simulink model "pend_slidingmode"  (Simulink 9.1)
settings: Solver=ode4  StartTime=0.0  StopTime=6  FixedStep=0.001  RelTol=1e-3  EnableMultiTasking=on
values from neighbouring files (symbols this model uses):
  a = J1 + m2*l1^2    (= 0.0264875)    [pend_lqr_init.m]
  b = m2*l1*l2    (= 0.001665)    [pend_lqr_init.m]
  c = m2*l2^2    (= 0.0016428)    [pend_lqr_init.m]
  c2 = 2.8*10^-3    (= 0.0028)    [pend_lqr_init.m]
  d = Kt*Ke/Ra + c1    (= 0.00529230769231)    [pend_lqr_init.m]
  f = J2 + m2*l2^2    (= 0.0055028)    [pend_lqr_init.m]
  h = m2*g*l2    (= 0.10878)    [pend_lqr_init.m]
settings Model: Creator=HOME  LastModifiedBy=DELL
settings DataIOCC: LimitDataPoints=on  SignalLoggingSaveFormat=ModelDataLogs
settings OptimizationCC: ExpressionDepthLimit=2147483647
settings DebuggingCC: SolverPrmCheckMsg=warning  FcnCallInpInsideContextMsg=warning  StateNameClashWarn=warning
settings GRTTargetCC: GeneratePreprocessorConditionals=Disable all

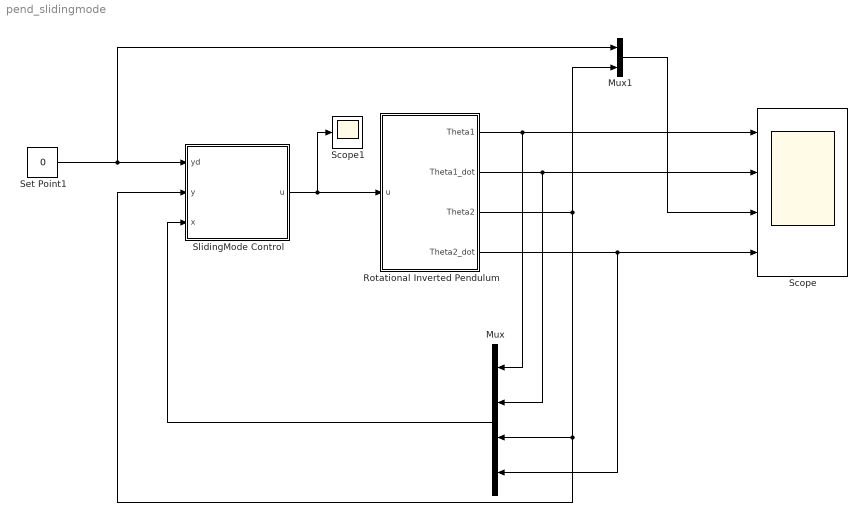
== system pend_slidingmode ==
  Mux : Mux
  Mux1 : Mux  Inputs=2
  Rotational Inverted Pendulum : Subsystem
  Scope : Scope  NumInputPorts=4
  Scope1 : Scope
  Set Point1 : Constant  Value=0
  SlidingMode Control : Subsystem
  wires:
  SlidingMode Control/1(u) -> Rotational Inverted Pendulum/1(u), Scope1/1
  Rotational Inverted Pendulum/1(Theta1) -> Scope/1, Mux/1
  Rotational Inverted Pendulum/2(Theta1_dot) -> Scope/2, Mux/2
  Rotational Inverted Pendulum/4(Theta2_dot) -> Scope/4, Mux/4
  Set Point1/1 -> Mux1/1, SlidingMode Control/1(yd)
  Rotational Inverted Pendulum/3(Theta2) -> Mux1/2, Mux/3, SlidingMode Control/2(y)
  Mux1/1 -> Scope/3
  Mux/1 -> SlidingMode Control/3(x)

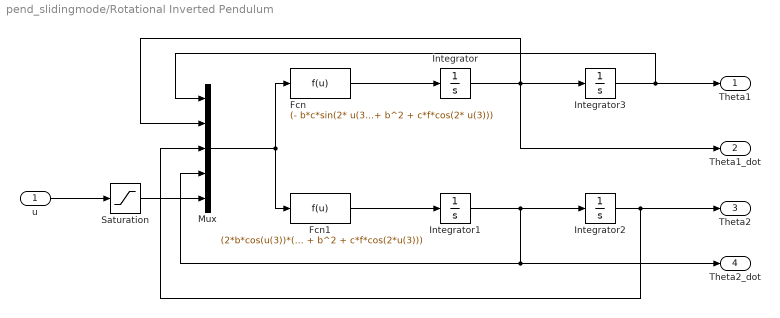
== system pend_slidingmode/Rotational Inverted Pendulum ==
  u : Inport
  Fcn : Fcn  Expr=(- b*c*sin(2* u(3))*cos(u(3))* u(2)^2 + 2*c*f*sin(2* u(3))* u(2)* u(4) + 2*d*f* u(2) + 2*b*f*sin(u(3))* u(4)^2 + 2*b*c2*cos(u(3))* u(4) - 2*e*f* u(5)- 2*b*h*cos(u(3))*sin(u(3)))/(b^2*cos(2* u(3)) - c*f - 2*a*f + b^2 + c*f*cos(2* u(3)))
  Fcn1 : Fcn  Expr=(2*b*cos(u(3))*(b*sin(u(3))*u(4)^2 + c*u(2)*sin(2*u(3))*u(4) + d*u(2) - e*u(5)))/(b^2*cos(2*u(3)) - c*f - 2*a*f + b^2 + c*f*cos(2*u(3))) - (((c*sin(2*u(3))*u(2)^2)/2 - c2*u(4) + h*sin(u(3)))*(2*a + c - c*cos(2*u(3))))/(b^2*cos(2*u(3)) - c*f - 2*a*f + b^2 + c*f*cos(2*u(3)))
  Integrator : Integrator
  Integrator1 : Integrator
  Integrator2 : Integrator  InitialCondition=15*pi/180
  Integrator3 : Integrator
  Mux : Mux  Inputs=5
  Saturation : Saturate  UpperLimit=25  LowerLimit=-25
  Theta1 : Outport
  Theta1_dot : Outport  Port=2
  Theta2 : Outport  Port=3
  Theta2_dot : Outport  Port=4
  wires:
  u/1 -> Saturation/1
  Saturation/1 -> Mux/5
  Mux/1 -> Fcn/1, Fcn1/1
  Fcn/1 -> Integrator/1
  Integrator/1 -> Integrator3/1, Theta1_dot/1, Mux/2
  Integrator3/1 -> Theta1/1, Mux/1
  Fcn1/1 -> Integrator1/1
  Integrator1/1 -> Integrator2/1, Theta2_dot/1, Mux/4
  Integrator2/1 -> Theta2/1, Mux/3

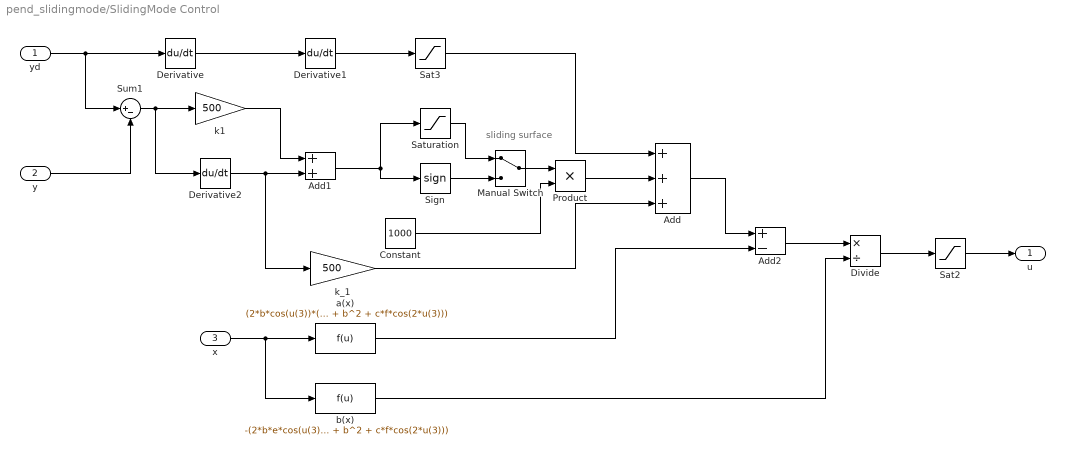
== system pend_slidingmode/SlidingMode Control ==
  note: sliding surface
  yd : Inport
  y : Inport  Port=2
  x : Inport  Port=3
  Add : Sum  Inputs=+++
  Add1 : Sum
  Add2 : Sum  Inputs=+-
  Constant : Constant  Value=1000
  Derivative : Derivative
  Derivative1 : Derivative
  Derivative2 : Derivative
  Divide : Product  Inputs=*/
  Manual Switch : ManualSwitch
  Product : Product  RndMeth=Zero
  Sat2 : Saturate  UpperLimit=25  LowerLimit=-25
  Sat3 : Saturate  UpperLimit=25  LowerLimit=-25
  Saturation : Saturate  UpperLimit=1  LowerLimit=-1
  Sign : Signum
  Sum1 : Sum  Inputs=|+-
  a(x) : Fcn  Expr=(2*b*cos(u(3))*(b*sin(u(3))*u(4)^2 + c*u(2)*sin(2*u(3))*u(4) + d*u(2) - e*0))/(b^2*cos(2*u(3)) - c*f - 2*a*f + b^2 + c*f*cos(2*u(3))) - (((c*sin(2*u(3))*u(2)^2)/2 - c2*u(4) + h*sin(u(3)))*(2*a + c - c*cos(2*u(3))))/(b^2*cos(2*u(3)) - c*f - 2*a*f + b^2 + c*f*cos(2*u(3)))
  b(x) : Fcn  Expr=-(2*b*e*cos(u(3)))/(b^2*cos(2*u(3)) - c*f - 2*a*f + b^2 + c*f*cos(2*u(3)))
  k1 : Gain  Gain=500
  k_1 : Gain  Gain=500
  u : Outport
  wires:
  yd/1 -> Derivative/1, Sum1/1
  Derivative/1 -> Derivative1/1
  Derivative1/1 -> Sat3/1
  Sum1/1 -> k1/1, Derivative2/1
  k1/1 -> Add1/1
  Derivative2/1 -> Add1/2, k_1/1
  y/1 -> Sum1/2
  Add1/1 -> Saturation/1, Sign/1
  Constant/1 -> Product/2
  Sat3/1 -> Add/1
  Product/1 -> Add/2
  k_1/1 -> Add/3
  x/1 -> a(x)/1, b(x)/1
  Add/1 -> Add2/1
  a(x)/1 -> Add2/2
  Add2/1 -> Divide/1
  b(x)/1 -> Divide/2
  Divide/1 -> Sat2/1
  Sat2/1 -> u/1
  Manual Switch/1 -> Product/1
  Sign/1 -> Manual Switch/2
  Saturation/1 -> Manual Switch/1
